simulink model "Final_System_Model_V10"  (R2018a)
settings: Solver=VariableStepAuto  StartTime=0  StopTime=250  FixedStep=0.5  RelTol=1e-3
PreLoadFcn:
  | Ts_Power=1e-6;
  | Ts_Control=100e-6;
undefined symbols (not defined in the file): DiscIntNeverNeededParam, sigbuilder_block
libraries: simulink x24, fl_lib x16, powerlib x15, nesl_utility x8, powerlib_meascontrol x5, re_lib x1
(part 2 of 8)

== system Final_System_Model_V10/Full System/Subsystem3/Battery ==
  Input current1 : Inport
  Batterytoload : Inport  Port=2
  Load Power (KW) : Inport  Port=3
  Input voltage1 : Inport  Port=4
  Battery1 : DiscreteIntegrator  IntegratorMethod=Accumulation: Forward Euler  gainval=1  InitialCondition=200  UpperSaturationLimit=100  LowerSaturationLimit=0  ICPrevOutput=DiscIntNeverNeededParam  ICPrevScaledInput=DiscIntNeverNeededParam
  Compare To Constant2 : simulink/Logic and Bit Operations/Compare To Constant  relop=>=  const=200  OutDataTypeStr=boolean
  Compare To Constant3 : simulink/Logic and Bit Operations/Compare To Constant  relop=<=  const=10  OutDataTypeStr=boolean
  Constant1 : Constant  Value=0.001
  Constant2 : Constant  Value=0
  Constant3 : Constant
  Gain1 : Gain  Gain=-1
  Gain2 : Gain  Gain=-1
  Gain3 : Gain  Gain=-1
  Product2 : Product  Inputs=3
  Switch1 : Switch  Criteria=u2 > Threshold
  Switch2 : Switch  Criteria=u2 > Threshold
  Switch3 : Switch  Criteria=u2 > Threshold
  Unit Delay : UnitDelay  SampleTime=-1
  Battery Full1 : Outport
  Battery Empty1 : Outport  Port=2
  Output Power (KW) : Outport  Port=3
  Input Power (KW) : Outport  Port=4
  wires:
  Input current1/1 -> Product2/1
  Input voltage1/1 -> Product2/2
  Product2/1 -> Gain3/1, Switch3/3  "Power(KW)"
  Constant1/1 -> Product2/3
  Compare To Constant2/1 -> Battery Full1/1, Switch1/2
  Constant2/1 -> Switch1/1
  Constant3/1 -> Switch1/3
  Compare To Constant3/1 -> Battery Empty1/1
  Batterytoload/1 -> Unit Delay/1
  Load Power (KW)/1 -> Gain1/1
  Switch2/1 -> Gain2/1, Switch3/1
  Gain1/1 -> Switch2/1
  Battery1/1 -> Compare To Constant2/1, Compare To Constant3/1
  Switch3/1 -> Battery1/1
  Gain2/1 -> Output Power (KW)/1
  Unit Delay/1 -> Switch3/2, Switch2/2
  Gain3/1 -> Input Power (KW)/1

== system Final_System_Model_V10/Full System/Subsystem3/DC-DC converter1 ==
  I in1 : Inport
  V in1 : Inport  Port=2
  V req1 : Inport  Port=3
  Divide : Product  Inputs=*/
  Product : Product
  Subsystem : Subsystem
  duty cycle : Subsystem
  V o : Outport
  I o : Outport  Port=2
  wires:
  [duty_cycle_battery] -> Subsystem/1(duty cycle)
  I in1/1 -> Product/1
  V in1/1 -> Product/2
  Product/1 -> Divide/1
  V req1/1 -> Divide/2, V o/1
  Divide/1 -> I o/1

== system Final_System_Model_V10/Full System/Subsystem3/Subsystem ==
  delta : Inport
  Fuel Cells Output (KW) : Inport  Port=2
  1st Mode : Subsystem
  2nd Mode : Subsystem
  5th Mode : Subsystem
  7th Mode : Subsystem
  Add1 : Sum  Inputs=++++
  Unit Delay{,1..3} (4 alike) : UnitDelay  SampleTime=-1
  Load to battery (KW) : Outport
  wires:
  delta/1 -> 1st Mode/1(delta), 2nd Mode/1(delta), 7th Mode/1(delta), 5th Mode/1(delta)
  Add1/1 -> Load to battery (KW)/1
  1st Mode/1(Load to battery (KW)) -> Unit Delay/1
  2nd Mode/1(Battery to load (KW)) -> Unit Delay1/1
  5th Mode/1(Battery to load (KW)) -> Unit Delay2/1
  7th Mode/1(Battery to load (KW)) -> Unit Delay3/1
  Unit Delay/1 -> Add1/1
  Unit Delay1/1 -> Add1/2
  Unit Delay2/1 -> Add1/3
  Unit Delay3/1 -> Add1/4
  Fuel Cells Output (KW)/1 -> 7th Mode/2(Fuel Cells Output (KW)), 5th Mode/2(Fuel Cells Output (KW)), 2nd Mode/2(Fuel Cells Output (KW)), 1st Mode/2(Fuel Cells Output (KW))

== system Final_System_Model_V10/Full System/Electrolysers/260 KW Electrolyzer Stack_1/electrolyser stack ==
  In1 : Inport
  In2 : Inport  Port=2
  Gain : Gain  Gain=2
  Multiply : Product
  Multiply1 : Product
  area in cm^2 : Constant  Value=428
  electrolyser cell : Subsystem
  number of cells : Constant  Value=212
  voltage : Scope
  Out1 : Outport
  Out3 : Outport  Port=2
  wires:
  area in cm^2/1 -> electrolyser cell/3(In3)
  Multiply/1 -> Out1/1
  number of cells/1 -> Multiply1/1, Multiply/1
  electrolyser cell/1(Out1) -> voltage/1, Multiply/2
  In1/1 -> electrolyser cell/1(In1)
  In2/1 -> electrolyser cell/2(In2)
  electrolyser cell/2(Out2) -> Gain/1
  Gain/1 -> Multiply1/2
  Multiply1/1 -> Out3/1

== system Final_System_Model_V10/Full System/Electrolysers/93 KW Electrolyzer Stack_2/electrolyser stack ==
  In1 : Inport
  In2 : Inport  Port=2
  Gain : Gain  Gain=2
  Multiply : Product
  Multiply1 : Product
  area in cm^2 : Constant  Value=428
  electrolyser cell : Subsystem
  number of cells : Constant  Value=212
  voltage : Scope
  Out1 : Outport
  Out3 : Outport  Port=2
  wires:
  Multiply1/1 -> Out3/1
  Gain/1 -> Multiply1/2
  electrolyser cell/2(Out2) -> Gain/1
  In2/1 -> electrolyser cell/2(In2)
  In1/1 -> electrolyser cell/1(In1)
  electrolyser cell/1(Out1) -> Multiply/2, voltage/1
  number of cells/1 -> Multiply/1, Multiply1/1
  Multiply/1 -> Out1/1
  area in cm^2/1 -> electrolyser cell/3(In3)

== system Final_System_Model_V10/Full System/Electrolysers/DC-DC converter/Subsystem ==
  duty cycle : Inport
  I in : Inport  Port=2
  V in : Inport  Port=3
  Constant : Constant
  I out : Product  Inputs=*/
  Multiply : Product
  Multiply1 : Product
  Subtract : Sum  Inputs=+-
  V out : Product  Inputs=*/
  efficiency : Gain  Gain=0.98
  efficiency1 : Gain  Gain=0.98
  I o : Outport
  V o : Outport  Port=2
  wires:
  Subtract/1 -> Multiply/1, V out/2
  efficiency/1 -> Multiply/2
  Multiply/1 -> I out/1
  Constant/1 -> Subtract/1
  duty cycle/1 -> Subtract/2, I out/2, Multiply1/2
  Multiply1/1 -> V out/1
  efficiency1/1 -> Multiply1/1
  I in/1 -> efficiency/1
  V out/1 -> V o/1
  I out/1 -> I o/1
  V in/1 -> efficiency1/1

== system Final_System_Model_V10/Full System/Electrolysers/DC-DC converter/duty cycle ==
  V in : Inport
  V req : Inport  Port=2
  Add : Sum
  Constant : Constant
  Divide : Product  Inputs=*/
  Gain : Gain  Gain=0.98
  Subtract : Sum  Inputs=+-
  tag scope: duty_cycle=global
  wires:
  Subtract/1 -> [duty_cycle]
  V req/1 -> Add/2
  V in/1 -> Gain/1
  Constant/1 -> Subtract/1
  Add/1 -> Divide/2
  Gain/1 -> Divide/1, Add/1
  Divide/1 -> Subtract/2

== system Final_System_Model_V10/Full System/Solar Panel + Solar Charge Controller/PV Insert inputs here/Signal Builder ==
  Demux : Demux  Tag=STV Demux  Outputs=1
  FromWs : FromWorkspace  Tag=STV FromWs  VariableName=tuvar  SampleTime=0
      SigBuilderData=|
      | common.afterFinalStr = 'Extrapolate'
      | common.sampleTime = 0
      | dataSet.timeRange = [0 300]
      | dataSet.name = 'Group 1'
      | sbobj.Groups.Name = 'Group 1'
      | sbobj.Groups.Signals.Name = 'Signal 1'
      | sbobj.Groups.Signals.XData = [0 1 2 3 4 5 6 7 8 9 10 11 12 13 14 15 16 17 18 19 20 21 22 23 24 25 26 27 28 29 30 31 32 33 34 35 36 37 38 39 40 41 42 43 44 45 46 47 48 49 50 51 52 53 54 55 56 57 58 59 60 61 62 63 64 65 66 67 68 69 70 71 72 73 74 75 76 77 78 79 80 81 82 83 84 85 86 87 88 89 90 91 92 93 94 95 96 97 98 99 100 101 102 103 104 105 106 107 108 109 110 111 112 113 114 115 116 117 118 119 120 121 122 123 124 125 126 127 128 129 130 131 132 133 134 135 136 137 138 139 140 141 142 143 144 145 146 147 148 149 150 151 152 153 154 155 156 157 158 159 160 161 162 163 164 165 166 167 168 169 170 171 172 173 174 175 176 177 178 179 180 181 182 183 184 185 186 187 188 189 190 191 192 193 194 195 196 197 198 199 200 201 202 203 204 205 206 207 208 209 210 211 212 213 214 215 216 217 218 219 220 221 222 223 224 225 226 227 228 229 230 231 232 233 234 235 236 237 238 300]
      | sbobj.Groups.Signals.YData = [0 0 0 0 0 0 0 150.811 439.714 763.14 970.278 1068.396 1081.115 979.363 770.408 481.505 172.615 0 0 0 0 0 0 0 0 0 0 0 0 0 0 167.164 486.956 815.833 1028.422 1124.723 1093.834 917.585 665.022 387.021 107.203 0 0 0 0 0 0 0 0 0 0 0 0 0 0 159.896 426.995 626.865 877.611 1124.723 1021.154 943.023 766.774 474.237 165.347 0 0 0 0 0 0 0 0 0 0 0 0 0 0 167.164 483.322 815.833 1033.873 1141.076 1151.978 1037.507 804.931 506.943 181.7 0 0 0 0 0 0 0 0 0 0 0 0 0 0 163.53 479.688 781.31 1002.984 1122.906 1121.089 1006.618 786.761 488.773 174.432 0 0 0 0 0 0 0 0 0 0 0 0 0 0 141.726 412.459 685.009 881.245 970.278 973.912 872.16 674.107 417.91 152.628 0 0 0 0 0 0 0 0 0 0 0 0 0 0 148.994 432.446 701.362 913.951 1032.056 1041.141 926.67 728.617 454.25 165.347 0 0 0 0 0 0 0 0 0 0 0 0 0 0 179.883 525.113 853.99 1099.285 1230.109 1233.743 1112.004 875.794 548.734 201.687 0 0 0 0 0 0 0 0 0 0 0 0 0 0 152.628 437.897 710.447 908.5 1010.252 997.533 904.866 712.264 452.433 168.981 0 0 0 0 0 0 0 0 0 0 0 0 0 0 159.896 470.603 784.944 1004.801 1153.795 1155.612 1055.677 837.637 521.479 188.968 1.817 0 0 0 0 0 0]
      | sbobj.Groups.TimeRange = [0 300]
  Signal 1 : Outport  Tag=STV Outport
  wires:
  Demux/1 -> Signal 1/1
  FromWs/1 -> Demux/1

== system Final_System_Model_V10/Full System/Solar Panel + Solar Charge Controller/PV Insert inputs here/Subsystem ==
  V_PV : Inport
  insolation : Inport  Port=2
  T_o : Inport  Port=3
  Rp : Inport  Port=4
  I_sc : Inport  Port=5
  Ns cells : Inport  Port=6
  V_oc : Inport  Port=7
  "C to K Converter " : Subsystem
  I o : Subsystem
  I on : Subsystem
  "I ph due to radiation " : Subsystem
  I pv : Subsystem
  NsAKt Thermal voltafe : Subsystem
  I_PV : Outport
  wires:
  T_o/1 -> "C to K Converter "/1(T_o)
  insolation/1 -> "I ph due to radiation "/1(insolation)
  "C to K Converter "/2(T_rk) -> I o/2(T_rk), "I ph due to radiation "/3(T_rk)  "T_nK"
  I_sc/1 -> "I ph due to radiation "/4(I_scn), I on/2(I_scn)  "I_scn"
  NsAKt Thermal voltafe/1(Ns*a*Kt) -> I pv/4(Ns*A*Kt1)  "const"
  I on/1(I_on) -> I o/3(I_on)  "I_on"
  "C to K Converter "/1(T_ak) -> "I ph due to radiation "/2(T_ak), I on/1(T_ref), I o/1(T_ak), NsAKt Thermal voltafe/1(T_ak T in kelven)  "T_ak"
  "I ph due to radiation "/1(I_photon) -> I pv/2(I_photon)  "I_ph"
  I pv/1(I_PV) -> I_PV/1
  I o/1(I_o) -> I pv/3(I_o)  "I_o"
  V_PV/1 -> I pv/1(V_PV)
  Rp/1 -> I pv/5(Rp Shunt resistance)
  Ns cells/1 -> I on/3(Num series)
  V_oc/1 -> I on/4(V_oc)

== system Final_System_Model_V10/Full System/Solar Panel + Solar Charge Controller/Solar Charge Controller/MPPT Controller using  "Incremental Conductance + Integral Regulator "  technique  ==
  V_PV : Inport
  I_PV : Inport  Port=2
  Add : Sum  Inputs=+-
  Deblock MPPT : Step  Time=0.4  SampleTime=0
  Duty Cycle : Constant  Value=Dinit
  MPPT : Subsystem
  PWM Generator (DC-DC) : powerlib_meascontrol/Pulse & Signal Generators/PWM Generator (DC-DC)  Fsw=fc  Ts=Ts_Power
  Saturation : Saturate  UpperLimit=1  LowerLimit=0
  Pulses : Outport
  wires:
  V_PV/1 -> MPPT/1(V_PV)
  I_PV/1 -> MPPT/2(I_PV)
  PWM Generator (DC-DC)/1 -> Pulses/1
  Deblock MPPT/1 -> MPPT/3(on/off)
  Saturation/1 -> PWM Generator (DC-DC)/1
  Add/1 -> Saturation/1  "D"
  MPPT/1(Delta_D) -> Add/2
  Duty Cycle/1 -> Add/1

== system Final_System_Model_V10/Full System/Solar Panel + Solar Charge Controller/Solar Charge Controller MPPT it is a device which track a point which has the max power/MPPT  ==
  note: P&O Algorism to track the max power point
  note: DC_DC Buck Boost Conveter
      |
      | to control the output Voltaage
  I_PV : Inport
  V_PV : Inport  Port=2
  Controlled Current Source : powerlib/Electrical Sources/Controlled Current Source  Initialize=on  Source_Type=DC  Amplitude=0  Phase=0  Frequency=0  Measurements=None
  DC Voltage Source : powerlib/Electrical Sources/DC Voltage Source  Amplitude=55  Measurements=None
  Diode : powerlib/Power Electronics/Diode  Ron=0.001  Lon=0  Vf=0.8  IC=0  UseSnubber=off  Rs=500  Cs=250e-9  Measurements=off
  Mosfet : powerlib/Power Electronics/Mosfet  Ron=0.001  Lon=0  Rd=0.01  Vfd=0  IC=0  Rs=1e5  Cs=inf  Measurements=off
  "P&O " : Subsystem
  Series RLC Branch : powerlib/Elements/Series RLC Branch  LConnTagsString=__new0  RConnTagsString=__new0  BranchType=RL  Resistance=.45  Inductance=1e-3  SetiL0=off  InitialCurrent=0  Capacitance=1e-6  Setx0=off  InitialVoltage=0  Measurements=None
  Series RLC Branch1 : powerlib/Elements/Series RLC Branch  LConnTagsString=__new0  RConnTagsString=__new0  BranchType=C  Resistance=1  Inductance=1e-3  SetiL0=off  InitialCurrent=0  Capacitance=2e-3  Setx0=off  InitialVoltage=0  Measurements=None
  Voltage Measurement : powerlib/Measurements/Voltage Measurement  PhasorSimulation=off  OutputType=Complex  PSBequivalent=0
  V_mpp : Outport
  wires:
  Voltage Measurement/1 -> V_mpp/1
  I_PV/1 -> "P&O "/1(I_pv), Controlled Current Source/1
  V_PV/1 -> "P&O "/2(V_PV)
  "P&O "/1(Signal) -> Mosfet/1
  connections:
  Series RLC Branch/RConn1 -- Mosfet/LConn1 -- Diode/LConn1
  Voltage Measurement/LConn1 -- Series RLC Branch/LConn1 -- Series RLC Branch1/LConn1 -- Controlled Current Source/RConn1
  Voltage Measurement/LConn2 -- DC Voltage Source/LConn1 -- Mosfet/RConn1 -- Series RLC Branch1/RConn1 -- Controlled Current Source/LConn1
  DC Voltage Source/RConn1 -- Diode/RConn1

== system Final_System_Model_V10/Full System/Subsystem1/100KW Fuel Cell Stack_2/From Load Current and Fuel Cell Output Current (A) to Valve Restriction Area (m^2) ==
  note: (3.0735e-14*(u(1)^3)) + (-5.0428e-11*(u(1)^2)) +(4.1772e-08*u(1)) + 2.7105e-07
  note: FEEDBACK BLOCK
  note: This block is the feedback block that controls the Flow control valve of the Hydrogen feeding system
      | I NPUTS: A) load Current (A) OUTPUTS: A) valve Restriction Area(m^2) as dictated by the Load Current
      | B) Output Current of the Fuel Cell (A) B) valve Restriction Area (m^2) as dictated by the Fuel Cell output current
  Load Profile Current (A) : Inport
  Output Current : Inport  Port=2
  Constant1 : Constant  Value=2.016e-3
  Constant2 : Constant  Value=96485
  Constant3 : Constant  Value=2
  Divide : Product  Inputs=*/
  Number Of Cells : Constant  Value=208
  Product : Product  Inputs=3
  Product1 : Product
  Subsystem : Subsystem
  Subsystem1 : Subsystem
  Valve Opening : Outport
  Valve Opening from Output Current : Outport  Port=2
  Hydrogen Mass Flow Rate (Kg/s) : Outport  Port=3
  wires:
  Output Current/1 -> Product/1, Subsystem/1(In1)
  Subsystem/1(Valve Opening from Output Current) -> Valve Opening from Output Current/1
  Load Profile Current (A)/1 -> Subsystem1/1(In1)
  Subsystem1/1(Out1) -> Valve Opening/1
  Product/1 -> Divide/1
  Number Of Cells/1 -> Product/2
  Constant1/1 -> Product/3
  Product1/1 -> Divide/2
  Constant3/1 -> Product1/2
  Constant2/1 -> Product1/1
  Divide/1 -> Hydrogen Mass Flow Rate (Kg/s)/1

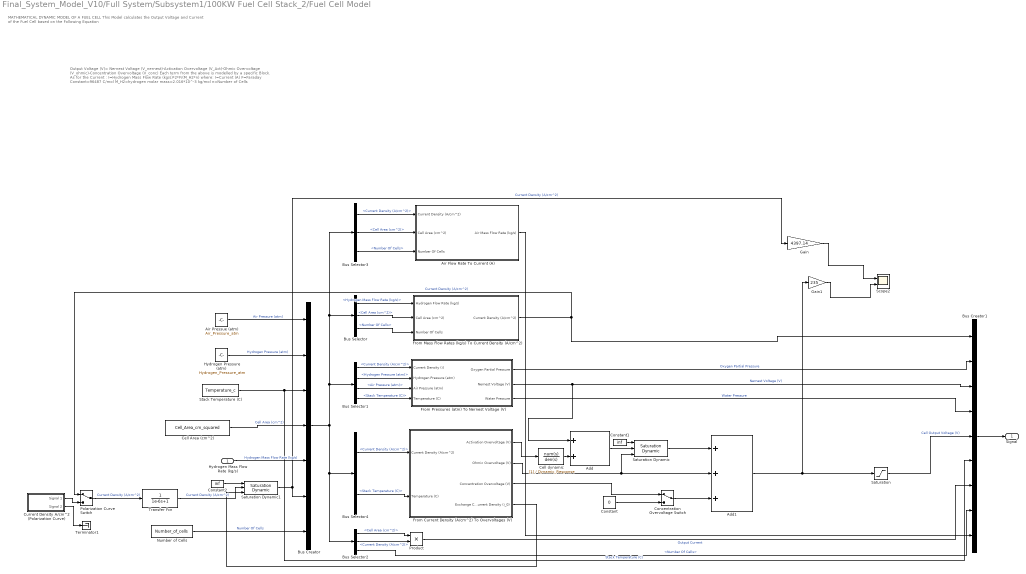
== system Final_System_Model_V10/Full System/Subsystem1/100KW Fuel Cell Stack_2/Fuel Cell Model ==
  note: Output Voltage (V)= Nernest Voltage (V_nernest)-Activation Overvoltage (V_Act)-Ohmic Overvoltage (V_ohmic)-Concentration Overvoltage (V_conc)
      | Each term from the above is modelled by a specific Block.
      | As for the Current :
      |
      | I=Hydrogen Mass Flow Rate (kg/s)*2*F/(M_H2*n)
      | where: I=Current (A)
      | F=Faraday Constant=96487 C/mol
      | M_H2=hydrogen molar mass=2.016*10^-3 kg/mol
      | n=Number of Cells
  note: MATHEMATICAL DYNAMIC MODEL OF A FUEL CELL
      | This Model calculates the Output Voltage and Current of the Fuel Cell based on the Following Equation
  Hydrogen Mass Flow Rate (kg/s) : Inport
  " From Current Density (A/cm^2) To Overvoltages (V)" : Subsystem
  Add : Sum
  Add1 : Sum  Inputs=+++
  Air Flow Rate To Current (A) : Subsystem
  Air Pressue (atm) : Constant  Value=Air_Pressure_atm
  Bus Creator : BusCreator  Inputs=7
  Bus Creator1 : BusCreator  Inputs=9
  Bus Selector : BusSelector  OutputSignals=Hydrogen Mass Flow Rate (kg/s),Cell Area (cm^2),Number Of Cells
  Bus Selector1 : BusSelector  OutputSignals=Current Density (A/cm^2),Hydrogen Pressure (atm),Air Pressure (atm),Stack Temperature (C)
  Bus Selector2 : BusSelector  OutputSignals=Cell Area (cm^2),Current Density (A/cm^2),Number Of Cells
  Bus Selector3 : BusSelector  OutputSignals=Current Density (A/cm^2),Cell Area (cm^2),Number Of Cells
  Bus Selector4 : BusSelector  OutputSignals=Current Density (A/cm^2),Stack Temperature (C)
  Cell Area (cm^2) : Constant  Value=Cell_Area_cm_squared
  Cell dynamic : TransferFcn  Denominator=Dynamic_Response
  Concentration Overvoltage Switch : ManualSwitch
  Constant : Constant  Value=0
  Constant1 : Constant  Value=inf
  Constant2 : Constant  Value=inf
  Current Density A/cm^2 (Polarization Curve) : Subsystem  Tag=STV Subsys  LoadFcn=sigbuilder_block('load');  StartFcn=sigbuilder_block('start');  StopFcn=sigbuilder_block('stop');  ClipboardFcn=sigbuilder_block('clipboard');  mask(Sigbuilder block){tuvar=[0:10]}
      mask help: Simulink:masks:SigbuilderBlock_MD
      mask init:
      | if ~strcmp(get_param(bdroot(gcbh),'SimulationStatus'),'stopped') tuvar = sigbuilder_block('maskInit'); end
      settings: CopyFcn=sigbuilder_block('copy');  DeleteFcn=sigbuilder_block('delete');  ModelCloseFcn=sigbuilder_block('modelClose');  PreSaveFcn=sigbuilder_block('preSave');  PauseFcn=sigbuilder_block('pause');  ContinueFcn=sigbuilder_block('continue');  NameChangeFcn=sigbuilder_block('namechange');  OpenFcn=sigbuilder_block('open',[403.5 117 550.5 359.25 ]);  CloseFcn=sigbuilder_block('close');
      mask Display: plot(0, 0, 100, 100,[2, 2, 32, 32, 2], [68, 8, 8, 68, 68],[32, 2], [38, 38], [32, 19, 2],[53, 60, 44], [32, 17, 17, 2],[16, 16, 31, 31]);txt = getActiveGroup(gcbh);text(2, 100, txt,'verticalAlignment', 'top');
  From Mass Flow Rates (kg/s) To Current Density (A/cm^2) : Subsystem
  From Pressures (atm) To Nernest Voltage (V) : Subsystem
  Gain : Gain  Gain=4397.14
  Gain1 : Gain  Gain=235
  Hydrogen Pressure (atm) : Constant  Value=Hydrogen_Pressure_atm
  Number of Cells : Constant  Value=Number_of_cells
  Polarization Curve Switch : ManualSwitch
  Product : Product
  Saturation : Saturate  UpperLimit=inf  LowerLimit=0  ZeroCross=off
  Saturation Dynamic : simulink/Discontinuities/Saturation Dynamic  OutMin=[]  OutMax=[]  OutDataTypeStr=Inherit: Same as second input  OutDataType=sfix(16)  OutScaling=2^-10  DoSatur=off
  Saturation Dynamic1 : simulink/Discontinuities/Saturation Dynamic  OutMin=[]  OutMax=[]  OutDataTypeStr=Inherit: Same as second input  OutDataType=sfix(16)  OutScaling=2^-10  DoSatur=off
  Scope2 : Scope  NumInputPorts=2
  Stack Temperature (C) : Constant  Value=Temperature_c
  Terminator1 : Terminator
  Transfer Fcn : TransferFcn  Denominator=[1e-6 1]
  Signal : Outport
  wires:
  Saturation/1 -> Bus Creator1/5  "Cell Output Voltage (V)"
  Current Density A/cm^2 (Polarization Curve)/1(Signal 1) -> Polarization Curve Switch/2
  Hydrogen Mass Flow Rate (kg/s)/1 -> Bus Creator/5  "Hydrogen Mass Flow Rate (kg/s)"
  Bus Creator/1 -> Bus Selector2/1, Bus Selector4/1, Bus Selector1/1, Bus Selector3/1, Bus Selector/1
  From Mass Flow Rates (kg/s) To Current Density (A/cm^2)/1(Current Density (A/cm^2)) -> Bus Creator1/1, Polarization Curve Switch/1  "Current Density (A/cm^2)"
  Bus Selector/1 -> From Mass Flow Rates (kg/s) To Current Density (A/cm^2)/1(Hydrogen Flow Rate (kg/s))  "<Hydrogen Mass Flow Rate (kg/s)>"
  Bus Selector/2 -> From Mass Flow Rates (kg/s) To Current Density (A/cm^2)/2(Cell Area (cm^2))  "<Cell Area (cm^2)>"
  From Pressures (atm) To Nernest Voltage (V)/2(Nernest Voltage (V)) -> Bus Creator1/3, Add/1  "Nernest Voltage (V)"
  Bus Selector1/1 -> From Pressures (atm) To Nernest Voltage (V)/1(Current Density (i))  "<Current Density (A/cm^2)>"
  Bus Selector1/2 -> From Pressures (atm) To Nernest Voltage (V)/2(Hydrogen Pressure (atm))  "<Hydrogen Pressure (atm)>"
  Bus Selector1/3 -> From Pressures (atm) To Nernest Voltage (V)/3(Air Pressure (atm))  "<Air Pressure (atm)>"
  Bus Selector1/4 -> From Pressures (atm) To Nernest Voltage (V)/4(Temperature (C))  "<Stack Temperature (C)>"
  From Pressures (atm) To Nernest Voltage (V)/1(Oxygen Partial Pressure) -> Bus Creator1/2  "Oxygen Partial Pressure"
  From Pressures (atm) To Nernest Voltage (V)/3(Water Pressure) -> Bus Creator1/4  "Water Pressure"
  Bus Selector4/1 -> " From Current Density (A/cm^2) To Overvoltages (V)"/1(Current Density (A/cm^2))  "<Current Density (A/cm^2)>"
  Bus Selector4/2 -> " From Current Density (A/cm^2) To Overvoltages (V)"/2(Temperature (C))  "<Stack Temperature (C)>"
  " From Current Density (A/cm^2) To Overvoltages (V)"/1(Activation Overvoltage (V)) -> Cell dynamic/1
  Bus Creator1/1 -> Signal/1
  Polarization Curve Switch/1 -> Transfer Fcn/1  "Current Density (A/cm^2)"
  Constant2/1 -> Saturation Dynamic1/1
  " From Current Density (A/cm^2) To Overvoltages (V)"/4(Exchange Current Density (i_0)) -> Saturation Dynamic1/3
  Add1/1 -> Gain1/1, Saturation/1
  Cell dynamic/1 -> Add/2
  Add/1 -> Saturation Dynamic/2
  Constant1/1 -> Saturation Dynamic/1
  Saturation Dynamic/1 -> Add1/1
  " From Current Density (A/cm^2) To Overvoltages (V)"/3(Concentration Overvoltage (V)) -> Concentration Overvoltage Switch/1
  Bus Selector2/2 -> Product/2  "<Current Density (A/cm^2)>"
  Bus Selector2/1 -> Product/1  "<Cell Area (cm^2)>"
  Product/1 -> Bus Creator1/7  "Output Current"
  Bus Selector/3 -> From Mass Flow Rates (kg/s) To Current Density (A/cm^2)/3(Number Of Cells)  "<Number Of Cells>"
  Bus Selector2/3 -> Bus Creator1/8  "<Number Of Cells>"
  Saturation Dynamic1/1 -> Bus Creator/6, Gain/1  "Current Density (A/cm^2)"
  Transfer Fcn/1 -> Saturation Dynamic1/2  "Current Density (A/cm^2)"
  Stack Temperature (C)/1 -> Bus Creator/3, Bus Creator1/6  "Stack Temperature (C)"
  Hydrogen Pressure (atm)/1 -> Bus Creator/2  "Hydrogen Pressure (atm)"
  Air Pressue (atm)/1 -> Bus Creator/1  "Air Pressure (atm)"
  Number of Cells/1 -> Bus Creator/7  "Number Of Cells"
  Cell Area (cm^2)/1 -> Bus Creator/4  "Cell Area (cm^2)"
  " From Current Density (A/cm^2) To Overvoltages (V)"/2(Ohmic Overvoltage (V)) -> Saturation Dynamic/3, Add1/2
  Concentration Overvoltage Switch/1 -> Add1/3
  Constant/1 -> Concentration Overvoltage Switch/2
  Air Flow Rate To Current (A)/1(Air Mass Flow Rate (kg/s)) -> Bus Creator1/9
  Current Density A/cm^2 (Polarization Curve)/2(Signal 2) -> Terminator1/1
  Gain/1 -> Scope2/1
  Gain1/1 -> Scope2/2
  Bus Selector3/1 -> Air Flow Rate To Current (A)/1(Current Density (A/cm^2))  "<Current Density (A/cm^2)>"
  Bus Selector3/2 -> Air Flow Rate To Current (A)/2(Cell Area (cm^2))  "<Cell Area (cm^2)>"
  Bus Selector3/3 -> Air Flow Rate To Current (A)/3(Number Of Cells)  "<Number Of Cells>"
